simulink model "testbench_straight"  (R2015a)
settings: Solver=ode45  StartTime=0.0  StopTime=10.0  RelTol=1e-3
libraries: legoev3lib x2
settings Model: Creator=USER  LastModifiedBy=USER

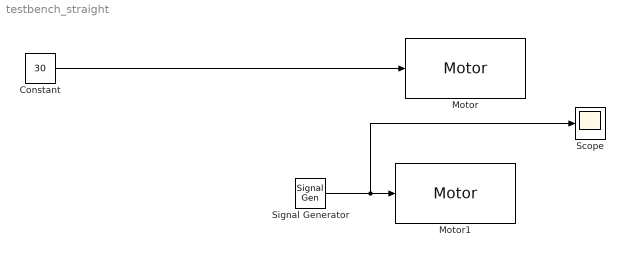
== system testbench_straight ==
  Constant : Constant  Value=30
  Motor : legoev3lib/Motor  sportNumber=A  sstopAction=Brake
  Motor1 : legoev3lib/Motor  sportNumber=B  sstopAction=Brake
  Scope : Scope
  Signal Generator : SignalGenerator  WaveForm=square  Frequency=50  Units=rad/sec
  wires:
  Constant/1 -> Motor/1
  Signal Generator/1 -> Scope/1, Motor1/1
